simulink model "ARI_09_pizza"  (Simulink 8.0)
settings: Solver=ode45  StartTime=0.0  StopTime=10.0  RelTol=1e-3
undefined symbols (not defined in the file or in its folder): A, B, C, D, sigbuilder_block
settings Model: Creator=Michael Sebek  ModifiedByFormat=Michael Sebek  LastModifiedBy=Michael Sebek
settings DataIOCC: SignalLoggingSaveFormat=ModelDataLogs
settings OptimizationCC: InitFltsAndDblsToZero=on
settings DebuggingCC: SaveWithParameterizedLinksMsg=none  SignalResolutionControl=TryResolveAllWithWarning  MultiTaskDSMMsg=warning  MultiTaskCondExecSysMsg=none  FcnCallInpInsideContextMsg=UseLocalSettings  StrictBusMsg=None
settings RTWCC: IncludeERTFirstTime=on
settings GRTTargetCC: TargetFcnLib=ansi_tfl_tmw.mat  CombineOutputUpdateFcns=off  GRTInterface=on

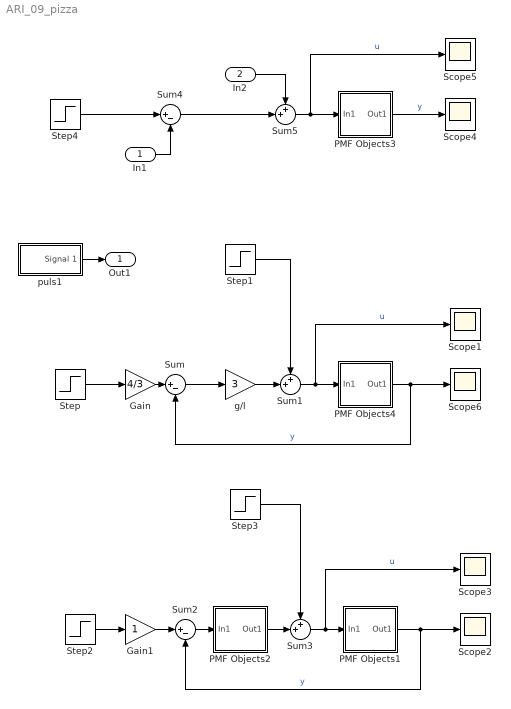
== system ARI_09_pizza ==
  In1 : Inport
  In2 : Inport  Port=2
  Gain : Gain  Gain=4/3
  Gain1 : Gain
  PMF Objects1 : Subsystem  mask(PMF Block){F=1/(s+1), InCon=[ ], SampTime=1, fvar=No change}
      mask prompts: F "PMF Object:"; InCon "Initial states:"; SampTime "Sample time (discrete time only):"; fvar "Force variable:"
      mask help:
      | Polynomial matrix fraction description of a linear system.
      |
      | This block represents a linear system defined by the polynomial matrix fraction of its transfer function.
      mask init:
      | Label = 'xxx';
      | [A,B,C,D,Label,var] = polymask2(F, fvar, length(InCon));
      | update;
      mask Help:
      | This block represents a linear system [<I>A,B,C,D</I>] defined by the polynomial matrix fraction (<I>PMF</I>) of its transfer function <I>T</I>.
      | <p>
      | <b>Left Matrix Fraction</b> item of the popup menu <b>Type</b> indicates the transfer function in the form of <I>left PMF</I>:
      | <p>
      | <I>T</I> = inv(<I>Q</I>) <I>P</I>.
      | <p>
      | <b>Right Matrix Fraction</b> item is used if the transfer function is given in the form of <I>right PMF</I>:
      | <p>
      | <I>T</I> = <I>P</I> inv(<I>Q</I>).
      | <p>
      |  The <b>variable</b> determines the type  of the system:
      | <p>
      | - <b>s, p</b> are used for continous time systems (Laplace transform).
      | <p>
      | - <b>z, q</b> are used for discrete time transfer functions in forward-shift operator (Z-transform).
      | <p>
      | - <b>d, z^-1</b> are used for discrete time transfer functions in backward-shift operator.
      | <p>
      | <b> Note:</b> For the variables <I>s,p,z,q</I>, the transfer function is defined as
      | <p>
      | <I>T</I> = <I>C</I> inv(<I>vI-A</I>) <I>B</I> + <I>D</I>,
      | <p>
      | where <I>v</I> is the variable of <I>P,Q</I>.
      | For the variables <I>d, z^-1</I>, the transfer function is defined as
      | <p>
      | <I>T</I> = <I>C v</I> inv(<I>I-Av</I>)  <I>B</I> + <I>D</I>.
      | <p>
      | <b>Note:</b> <b>Initial states</b> concern the observer-form realization of the system as defined by LMF2S and RMF2S functions. Their number must equal the sum of column degrees of the denominator matrix <I>Q</I> in case of right PMF and the sum of row degrees of <I>Q</I> for left PMF description.
      | <p>
      | See also POL, LMF2S, RMF2S.
      mask TypeOptions fvar: No change | s   (continous time) | p   (continous time) | z      (discrete time) | q      (discrete time) | d      (discrete time) | z^-1 (discrete time)
      mask Display: image(imread('PecNaPizzu.jpg'))
  PMF Objects2 : Subsystem  mask(PMF Block){F=7+16/s, InCon=[ ], SampTime=1, fvar=No change}
      mask prompts: F "PMF Object:"; InCon "Initial states:"; SampTime "Sample time (discrete time only):"; fvar "Force variable:"
      mask help:
      | Polynomial matrix fraction description of a linear system.
      |
      | This block represents a linear system defined by the polynomial matrix fraction of its transfer function.
      mask init:
      | Label = 'xxx';
      | [A,B,C,D,Label,var] = polymask2(F, fvar, length(InCon));
      | update;
      mask Help:
      | This block represents a linear system [<I>A,B,C,D</I>] defined by the polynomial matrix fraction (<I>PMF</I>) of its transfer function <I>T</I>.
      | <p>
      | <b>Left Matrix Fraction</b> item of the popup menu <b>Type</b> indicates the transfer function in the form of <I>left PMF</I>:
      | <p>
      | <I>T</I> = inv(<I>Q</I>) <I>P</I>.
      | <p>
      | <b>Right Matrix Fraction</b> item is used if the transfer function is given in the form of <I>right PMF</I>:
      | <p>
      | <I>T</I> = <I>P</I> inv(<I>Q</I>).
      | <p>
      |  The <b>variable</b> determines the type  of the system:
      | <p>
      | - <b>s, p</b> are used for continous time systems (Laplace transform).
      | <p>
      | - <b>z, q</b> are used for discrete time transfer functions in forward-shift operator (Z-transform).
      | <p>
      | - <b>d, z^-1</b> are used for discrete time transfer functions in backward-shift operator.
      | <p>
      | <b> Note:</b> For the variables <I>s,p,z,q</I>, the transfer function is defined as
      | <p>
      | <I>T</I> = <I>C</I> inv(<I>vI-A</I>) <I>B</I> + <I>D</I>,
      | <p>
      | where <I>v</I> is the variable of <I>P,Q</I>.
      | For the variables <I>d, z^-1</I>, the transfer function is defined as
      | <p>
      | <I>T</I> = <I>C v</I> inv(<I>I-Av</I>)  <I>B</I> + <I>D</I>.
      | <p>
      | <b>Note:</b> <b>Initial states</b> concern the observer-form realization of the system as defined by LMF2S and RMF2S functions. Their number must equal the sum of column degrees of the denominator matrix <I>Q</I> in case of right PMF and the sum of row degrees of <I>Q</I> for left PMF description.
      | <p>
      | See also POL, LMF2S, RMF2S.
      mask TypeOptions fvar: No change | s   (continous time) | p   (continous time) | z      (discrete time) | q      (discrete time) | d      (discrete time) | z^-1 (discrete time)
      mask Display: disp(Label);
  PMF Objects3 : Subsystem  mask(PMF Block){F=1/(s+1), InCon=[ ], SampTime=1, fvar=No change}
      mask prompts: F "PMF Object:"; InCon "Initial states:"; SampTime "Sample time (discrete time only):"; fvar "Force variable:"
      mask help:
      | Polynomial matrix fraction description of a linear system.
      |
      | This block represents a linear system defined by the polynomial matrix fraction of its transfer function.
      mask init:
      | Label = 'xxx';
      | [A,B,C,D,Label,var] = polymask2(F, fvar, length(InCon));
      | update;
      mask Help:
      | This block represents a linear system [<I>A,B,C,D</I>] defined by the polynomial matrix fraction (<I>PMF</I>) of its transfer function <I>T</I>.
      | <p>
      | <b>Left Matrix Fraction</b> item of the popup menu <b>Type</b> indicates the transfer function in the form of <I>left PMF</I>:
      | <p>
      | <I>T</I> = inv(<I>Q</I>) <I>P</I>.
      | <p>
      | <b>Right Matrix Fraction</b> item is used if the transfer function is given in the form of <I>right PMF</I>:
      | <p>
      | <I>T</I> = <I>P</I> inv(<I>Q</I>).
      | <p>
      |  The <b>variable</b> determines the type  of the system:
      | <p>
      | - <b>s, p</b> are used for continous time systems (Laplace transform).
      | <p>
      | - <b>z, q</b> are used for discrete time transfer functions in forward-shift operator (Z-transform).
      | <p>
      | - <b>d, z^-1</b> are used for discrete time transfer functions in backward-shift operator.
      | <p>
      | <b> Note:</b> For the variables <I>s,p,z,q</I>, the transfer function is defined as
      | <p>
      | <I>T</I> = <I>C</I> inv(<I>vI-A</I>) <I>B</I> + <I>D</I>,
      | <p>
      | where <I>v</I> is the variable of <I>P,Q</I>.
      | For the variables <I>d, z^-1</I>, the transfer function is defined as
      | <p>
      | <I>T</I> = <I>C v</I> inv(<I>I-Av</I>)  <I>B</I> + <I>D</I>.
      | <p>
      | <b>Note:</b> <b>Initial states</b> concern the observer-form realization of the system as defined by LMF2S and RMF2S functions. Their number must equal the sum of column degrees of the denominator matrix <I>Q</I> in case of right PMF and the sum of row degrees of <I>Q</I> for left PMF description.
      | <p>
      | See also POL, LMF2S, RMF2S.
      mask TypeOptions fvar: No change | s   (continous time) | p   (continous time) | z      (discrete time) | q      (discrete time) | d      (discrete time) | z^-1 (discrete time)
      mask Display: image(imread('PecNaPizzu.jpg'))
  PMF Objects4 : Subsystem  mask(PMF Block){F=1/(s+1), InCon=[ ], SampTime=1, fvar=No change}
      mask prompts: F "PMF Object:"; InCon "Initial states:"; SampTime "Sample time (discrete time only):"; fvar "Force variable:"
      mask help:
      | Polynomial matrix fraction description of a linear system.
      |
      | This block represents a linear system defined by the polynomial matrix fraction of its transfer function.
      mask init:
      | Label = 'xxx';
      | [A,B,C,D,Label,var] = polymask2(F, fvar, length(InCon));
      | update;
      mask Help:
      | This block represents a linear system [<I>A,B,C,D</I>] defined by the polynomial matrix fraction (<I>PMF</I>) of its transfer function <I>T</I>.
      | <p>
      | <b>Left Matrix Fraction</b> item of the popup menu <b>Type</b> indicates the transfer function in the form of <I>left PMF</I>:
      | <p>
      | <I>T</I> = inv(<I>Q</I>) <I>P</I>.
      | <p>
      | <b>Right Matrix Fraction</b> item is used if the transfer function is given in the form of <I>right PMF</I>:
      | <p>
      | <I>T</I> = <I>P</I> inv(<I>Q</I>).
      | <p>
      |  The <b>variable</b> determines the type  of the system:
      | <p>
      | - <b>s, p</b> are used for continous time systems (Laplace transform).
      | <p>
      | - <b>z, q</b> are used for discrete time transfer functions in forward-shift operator (Z-transform).
      | <p>
      | - <b>d, z^-1</b> are used for discrete time transfer functions in backward-shift operator.
      | <p>
      | <b> Note:</b> For the variables <I>s,p,z,q</I>, the transfer function is defined as
      | <p>
      | <I>T</I> = <I>C</I> inv(<I>vI-A</I>) <I>B</I> + <I>D</I>,
      | <p>
      | where <I>v</I> is the variable of <I>P,Q</I>.
      | For the variables <I>d, z^-1</I>, the transfer function is defined as
      | <p>
      | <I>T</I> = <I>C v</I> inv(<I>I-Av</I>)  <I>B</I> + <I>D</I>.
      | <p>
      | <b>Note:</b> <b>Initial states</b> concern the observer-form realization of the system as defined by LMF2S and RMF2S functions. Their number must equal the sum of column degrees of the denominator matrix <I>Q</I> in case of right PMF and the sum of row degrees of <I>Q</I> for left PMF description.
      | <p>
      | See also POL, LMF2S, RMF2S.
      mask TypeOptions fvar: No change | s   (continous time) | p   (continous time) | z      (discrete time) | q      (discrete time) | d      (discrete time) | z^-1 (discrete time)
      mask Display: image(imread('PecNaPizzu.jpg'))
  Scope{1..6} (6 alike) : Scope
      Scope2 settings: SaveName=ScopeData2
      Scope3 settings: SaveName=ScopeData3
      Scope4 settings: SaveName=ScopeData4
      Scope5 settings: SaveName=ScopeData5
  Step : Step  Time=0  SampleTime=0
  Step1 : Step  Time=5  After=-1  SampleTime=0
  Step2 : Step  Time=0  SampleTime=0
  Step3 : Step  Time=5  After=-1  SampleTime=0
  Step4 : Step  Time=0  SampleTime=0
  Sum : Sum  Inputs=|+-
  Sum1 : Sum  Inputs=++|
  Sum2 : Sum  Inputs=|+-
  Sum3 : Sum  Inputs=++|
  Sum4 : Sum  Inputs=|+-
  Sum5 : Sum  Inputs=++|
  g/l : Gain  Gain=3
  puls1 : Subsystem  Tag=STV Subsys  LoadFcn=sigbuilder_block('load');  StartFcn=sigbuilder_block('start');  StopFcn=sigbuilder_block('stop');  ClipboardFcn=sigbuilder_block('clipboard');  mask(Sigbuilder block){}
      mask help: Sigbuilder GUI
      mask init:
      | if ~strcmp(get_param(bdroot(gcbh),'SimulationStatus'),'stopped') tuvar = sigbuilder_block('maskInit'); end
      settings: CopyFcn=sigbuilder_block('copy');  DeleteFcn=sigbuilder_block('delete');  ModelCloseFcn=sigbuilder_block('modelClose');  PreSaveFcn=sigbuilder_block('preSave');  PauseFcn=sigbuilder_block('pause')  ContinueFcn=sigbuilder_block('continue')  NameChangeFcn=sigbuilder_block('namechange');  OpenFcn=sigbuilder_block('open',[437.6 199.2 550.4 400 ]);  CloseFcn=sigbuilder_block('close');
      mask Display: plot(0,0,100,100,[10,10,40,40,10],[80,20,20,80,80],[40,10],[50,50], [40,27,10],[65,72,56],[40,25,25,10],[28,28,43,43]);
  Out1 : Outport
  wires:
  Sum1/1 -> Scope1/1, PMF Objects4/1(In1)  "u"
  PMF Objects4/1(Out1) -> Sum/2, Scope6/1  "y"
  Step/1 -> Gain/1
  Sum/1 -> g/l/1
  Gain/1 -> Sum/1
  g/l/1 -> Sum1/2
  Step1/1 -> Sum1/1
  Sum3/1 -> PMF Objects1/1(In1), Scope3/1  "u"
  PMF Objects1/1(Out1) -> Scope2/1, Sum2/2  "y"
  Step2/1 -> Gain1/1
  Gain1/1 -> Sum2/1
  PMF Objects2/1(Out1) -> Sum3/2
  Step3/1 -> Sum3/1
  Sum2/1 -> PMF Objects2/1(In1)
  Sum5/1 -> Scope5/1, PMF Objects3/1(In1)  "u"
  PMF Objects3/1(Out1) -> Scope4/1  "y"
  Step4/1 -> Sum4/1
  Sum4/1 -> Sum5/2
  In1/1 -> Sum4/2
  In2/1 -> Sum5/1
  puls1/1(Signal 1) -> Out1/1

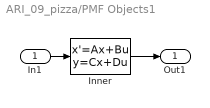
== system ARI_09_pizza/PMF Objects1 ==
  In1 : Inport
  Inner : StateSpace  A=A  B=B  C=C  D=D  X0=InCon
  Out1 : Outport
  wires:
  Inner/1 -> Out1/1
  In1/1 -> Inner/1

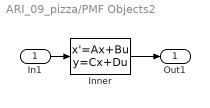
== system ARI_09_pizza/PMF Objects2 ==
  In1 : Inport
  Inner : StateSpace  A=A  B=B  C=C  D=D  X0=InCon
  Out1 : Outport
  wires:
  Inner/1 -> Out1/1
  In1/1 -> Inner/1

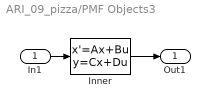
== system ARI_09_pizza/PMF Objects3 ==
  In1 : Inport
  Inner : StateSpace  A=A  B=B  C=C  D=D  X0=InCon
  Out1 : Outport
  wires:
  In1/1 -> Inner/1
  Inner/1 -> Out1/1

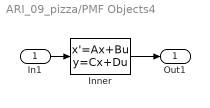
== system ARI_09_pizza/PMF Objects4 ==
  In1 : Inport
  Inner : StateSpace  A=A  B=B  C=C  D=D  X0=InCon
  Out1 : Outport
  wires:
  In1/1 -> Inner/1
  Inner/1 -> Out1/1

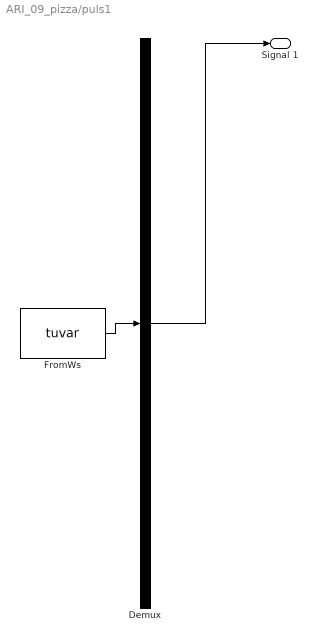
== system ARI_09_pizza/puls1 ==
  Demux : Demux  Tag=STV Demux  Outputs=1
  FromWs : FromWorkspace  Tag=STV FromWs  VariableName=tuvar  SampleTime=0  SigBuilderData=DataTag0  VnvData=DataTag1
      SigBuilderData=|
      | common.afterFinalStr = 'Extrapolate'
      | common.sampleTime = 0
      | dataSet.timeRange = [0 10]
      | dataSet.name = 'Group 1'
      | sbobj.Groups.Name = 'Group 1'
      | sbobj.Groups.Signals.Name = 'Signal 1'
      | sbobj.Groups.Signals.XData = [0 4 4 6 6 10]
      | sbobj.Groups.Signals.YData = [0 0 1 1 0 0]
  Signal 1 : Outport  Tag=STV Outport
  wires:
  Demux/1 -> Signal 1/1
  FromWs/1 -> Demux/1
